simulink model "EKF"  (R2023a)
settings: Solver=VariableStepAuto  StartTime=0.0  StopTime=10.0  RelTol=1e-3
settings Model: Creator=belov  LastModifiedBy=belov

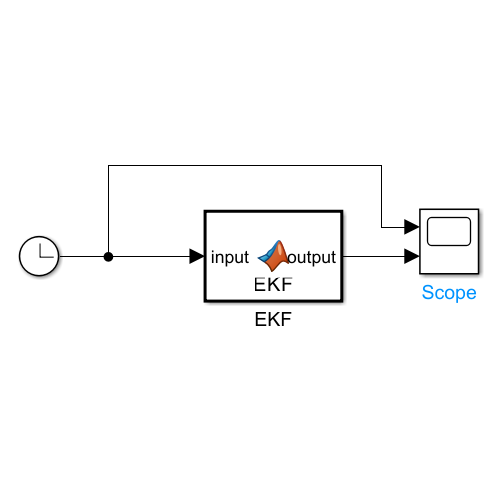
[thumbnail: Simulink's stored preview of the top-level diagram]
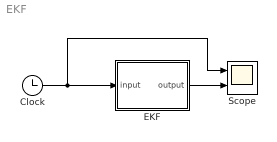
== system EKF ==
  Clock : Clock
  EKF : MATLAB Function  TreatAsAtomicUnit=on
  Scope : Scope  NumInputPorts=2
  wires:
  Clock/1 -> Scope/1, EKF/1(input)
  EKF/1(output) -> Scope/2

== matlab function EKF/EKF ==
  data: input input; output output
function output = EKF(input)


persistent x_last_last P_last_last;
if(isempty(x_last_last))
    x_last_last = 0;
end
if(isempty(P_last_last))
    P_last_last = 1;
end

F_k = 1;
Q_k = 1;
R_k = 0.01;

x_last_now = F_k * x_last_last;

% JF = jacobian(x_last_now, x_last_last);
JF = 1;
%%%% 这里应该对上式求雅各比矩阵，对于一个复杂的系统来说，X 应当是一个多维度的矩阵

P_last_now = JF * P_last_last * JF' + Q_k;

H_k = 1;

% JH = jacobian(H_k * x_last_now, x_last_now);
JH = 1;

y_k = input - x_last_now;
S_k = JH * P_last_now * JH' + R_k;
K_k = P_last_now * JH' * inv(S_k);
x_now_now = x_last_now + K_k * y_k;

I = eye(size(K_k * JH));
P_now_now = (I - K_k * JH) * P_last_now;

P_last_last = P_now_now;
x_last_last = x_now_now;

output = x_now_now;
